simulink model "Modelper"  (Simulink 8.5)
settings: Solver=ode45  StartTime=0.0  StopTime=0.1  RelTol=1e-3
undefined symbols (not defined in the file or in its folder): u1per, u2per, x01per, x02per
settings Model: Creator=Default  LastModifiedBy=Default
settings DataIOCC: SignalLoggingSaveFormat=Dataset
settings OptimizationCC: ExpressionDepthLimit=128
settings DebuggingCC: UnderspecifiedInitializationDetection=Simplified  MergeDetectMultiDrivingBlocksExec=error  FcnCallInpInsideContextMsg=EnableAllAsError  StateNameClashWarn=none
settings GRTTargetCC: CombineOutputUpdateFcns=on  GRTInterface=off

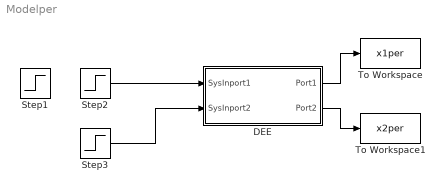
== system Modelper ==
  DEE : Subsystem  mask(Differential Equation Editor (DEE)){}
      settings: OpenFcn=diffeqed
      mask Display: disp('Differential Equation\n Editor')
  Step1 : Step  Time=0  After=u1per  SampleTime=0
  Step2 : Step  Time=0  After=u1per  SampleTime=0
  Step3 : Step  Time=0  After=u2per  SampleTime=0
  To Workspace : ToWorkspace  VariableName=x1per  SampleTime=-1
  To Workspace1 : ToWorkspace  VariableName=x2per  SampleTime=-1
  wires:
  Step2/1 -> DEE/1(SysInport1)
  DEE/1(Port1) -> To Workspace/1
  DEE/2(Port2) -> To Workspace1/1
  Step3/1 -> DEE/2(SysInport2)

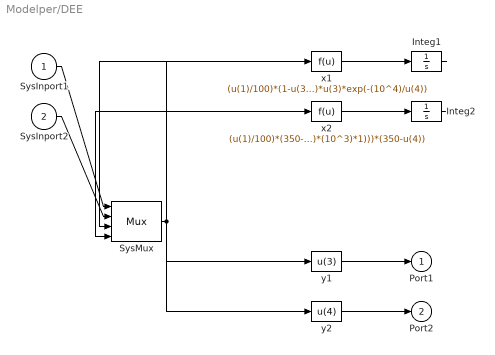
== system Modelper/DEE ==
  SysInport1 : Inport
  SysInport2 : Inport  Port=2
  Integ1 : Integrator  InitialCondition=x01per
  Integ2 : Integrator  InitialCondition=x02per
  SysMux : Mux
  x1 : Fcn  Expr=(u(1)/100)*(1-u(3))-(7.2*10^10)*u(3)*exp(-(10^4)/u(4))
  x2 : Fcn  Expr=(u(1)/100)*(350-u(4))-((-(2*10^5)/(10^3))*(7.2*10^10)*u(3)*exp(-(10^4)/u(4)))+(((10^3)*1)/((10^3)*100))*(u(2))*(1-exp(-(7*10^5)/(u(2)*(10^3)*1)))*(350-u(4))
  y1 : Fcn  Expr=u(3)
  y2 : Fcn  Expr=u(4)
  Port1 : Outport
  Port2 : Outport  Port=2
  wires:
  SysInport1/1 -> SysMux/1
  SysInport2/1 -> SysMux/2
  SysMux/1 -> x1/1, x2/1, y1/1, y2/1
  x1/1 -> Integ1/1
  Integ1/1 -> SysMux/3
  x2/1 -> Integ2/1
  Integ2/1 -> SysMux/4
  y1/1 -> Port1/1
  y2/1 -> Port2/1
